simulink model "int2bit"  (Simulink 8.1)
settings: Solver=ode45  StartTime=0.0  StopTime=10  FixedStep=1/500000  RelTol=1e-3
CloseFcn:
  | rtwprivate ssgencode ModelCloseRequest untitled
settings Model: Creator=Administrator  LastModifiedBy=cell
settings OptimizationCC: ExpressionDepthLimit=128  InitFltsAndDblsToZero=on
settings DebuggingCC: SaveWithParameterizedLinksMsg=none  SignalResolutionControl=TryResolveAllWithWarning  SolverPrmCheckMsg=none  MultiTaskDSMMsg=warning  MultiTaskCondExecSysMsg=none  FcnCallInpInsideContextMsg=EnableAllAsError  StrictBusMsg=None
settings HardwareCC: TargetUnknown=on
settings RTWCC: IncludeERTFirstTime=on
settings GRTTargetCC: TargetFcnLib=ansi_tfl_tmw.mat

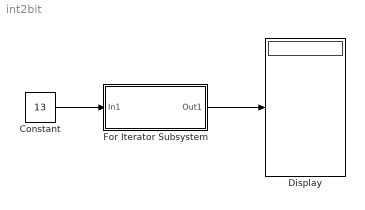
== system int2bit ==
  Constant : Constant  Value=13  OutDataTypeStr=uint8  SampleTime=1/10
  Display : Display
  For Iterator Subsystem : Subsystem  TreatAsAtomicUnit=on  mask{bits=8}
      mask prompts: bits "ビット数"
      mask Display: disp('Integer To Bit\nConvertor')
  wires:
  Constant/1 -> For Iterator Subsystem/1(In1)
  For Iterator Subsystem/1(Out1) -> Display/1

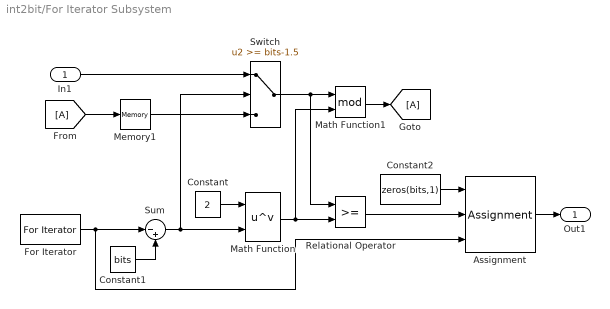
== system int2bit/For Iterator Subsystem ==
  In1 : Inport
  Assignment : Assignment  IndexOptions=Index vector (port)  Indices=1  OutputSizes=[1 1]
  Constant : Constant  Value=2
  Constant1 : Constant  Value=bits
  Constant2 : Constant  Value=zeros(bits,1)  VectorParams1D=off
  For Iterator : ForIterator  IterationLimit=bits
  Math Function : Math  Operator=pow  SaturateOnIntegerOverflow=on
  Math Function1 : Math  Operator=mod  SaturateOnIntegerOverflow=on
  Memory1 : Memory  InheritSampleTime=on
  Relational Operator : RelationalOperator  OutDataTypeStr=float('double')
  Sum : Sum  Inputs=|-+
  Switch : Switch  Threshold=bits-1.5
  Out1 : Outport
  wires:
  For Iterator/1 -> Sum/1, Assignment/3
  Constant/1 -> Math Function/1
  Sum/1 -> Math Function/2, Switch/2
  Constant1/1 -> Sum/2
  Math Function/1 -> Math Function1/2, Relational Operator/2
  Switch/1 -> Math Function1/1, Relational Operator/1
  In1/1 -> Switch/1
  Memory1/1 -> Switch/3
  Assignment/1 -> Out1/1
  Constant2/1 -> Assignment/1
  Relational Operator/1 -> Assignment/2
  [A] -> Memory1/1
  Math Function1/1 -> [A]
